simulink model "RealTime_model"  (R2015b)
settings: Solver=FixedStepAuto  StartTime=0.0  StopTime=tFinal  FixedStep=T  RelTol=1e-3
values from neighbouring files (symbols this model uses):
  PulseAmplitude = 2    [MAIN_RealTime.m]
  PulsePeriod = 1    [MAIN_RealTime.m]
  PulseWidth = 25    [MAIN_RealTime.m]
libraries: UWArduinoBlockset_Due x1
settings Model: SimulationMode=external  ExtModeTrigDuration=5000  Creator=Christopher  LastModifiedBy=Christopher
settings DataIOCC: StreamToWorkspace=on
settings OptimizationCC: OptimizeModelRefInitCode=on  LifeSpan=1  MaxStackSize=64
settings HardwareCC: ProdBitPerPointer=32  ProdLargestAtomicInteger=Long  ProdLargestAtomicFloat=Double  ProdWordSize=32  ProdHWDeviceType=ARM Compatible->ARM Cortex
settings RTWCC: SystemTargetFile=ert.tlc  TemplateMakefile=ert_default_tmf  Description=Embedded Coder  Toolchain=Arduino ARM v1.6.1  BuildConfiguration=Faster Runs
settings CodeAppCC: IgnoreCustomStorageClasses=off
settings ERTTargetCC: SupportContinuousTime=on  SupportVariableSizeSignals=on

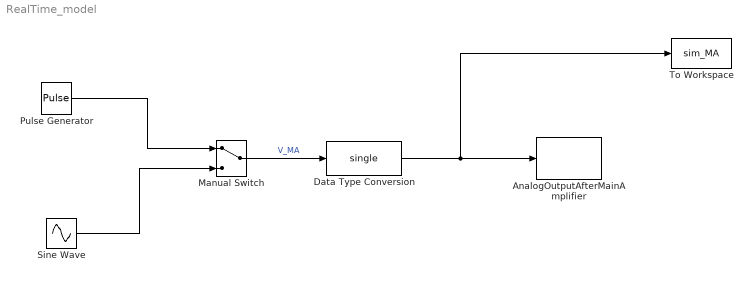
== system RealTime_model ==
  AnalogOutputAfterMainAmplifier : UWArduinoBlockset_Due/AnalogOutputAfterMainAmplifier  K_preamp=K_preamp  K_kepco=K_kepco
  Data Type Conversion : DataTypeConversion  OutDataTypeStr=single
  Manual Switch : ManualSwitch
  Pulse Generator : DiscretePulseGenerator  PulseType=Time based  Amplitude=PulseAmplitude  Period=PulsePeriod  PulseWidth=PulseWidth
  Sine Wave : Sin  Amplitude=20  Frequency=5  SampleTime=0
  To Workspace : ToWorkspace  VariableName=sim_MA  SaveFormat=Structure With Time  SampleTime=-1
  wires:
  Manual Switch/1 -> Data Type Conversion/1  "V_MA"
  Pulse Generator/1 -> Manual Switch/1
  Sine Wave/1 -> Manual Switch/2
  Data Type Conversion/1 -> AnalogOutputAfterMainAmplifier/1, To Workspace/1
